simulink model "lqgd_mdl"  (Simulink 5.0)
settings: Solver=ode23s  StartTime=0.0  StopTime=200  RelTol=1e-8  AbsTol=1e-8
values from neighbouring files (symbols this model uses):
  A = [1 -0.9]    [lqg_as1.m]    (also in lqg_ex.m = [1 -0.44]; spec_ex.m = conv([-0.5 1],[-0.9 1]); specfac_ex.m = conv([1 -1],[1 -0.9]))
  B = [0.1 0.08]    [lqg_as1.m]    (also in lqg_ex.m = [0.51 1.21]; lqg_pend.m = num(first_nz:length(num)); spec_ex.m = 0.5*[-0.9 1]; specfac_ex.m)
  C = 1    [lqg_as1.m]    (also in lqg_ex.m = A; lqg_pend.m = A; specfac_ex.m = zeros(1,2))
  Ts = 0.01    [lqg_pend.m]
undefined symbols (not defined in the file or in its folder): R, S, zk
settings Model: Creator=kannanm  LastModifiedBy=kannan  ExtModeAutoUpdateStatusClock=off

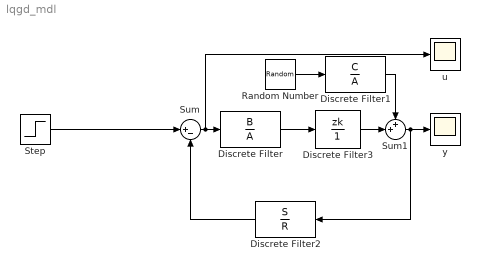
== system lqgd_mdl ==
  Discrete Filter : DiscreteFilter  Numerator=B  Denominator=A  SampleTime=Ts
  Discrete Filter1 : DiscreteFilter  Numerator=C  Denominator=A  SampleTime=Ts
  Discrete Filter2 : DiscreteFilter  Orientation=left  Numerator=S  Denominator=R  SampleTime=Ts
  Discrete Filter3 : DiscreteFilter  Numerator=zk  Denominator=1  SampleTime=Ts
  Random Number : RandomNumber  Variance=0.01  SampleTime=Ts
  Step : Step  After=0  SampleTime=Ts
  Sum : Sum  Inputs=|+-  SaturateOnIntegerOverflow=on
  Sum1 : Sum  Inputs=++|  SaturateOnIntegerOverflow=on
  u : Scope
  y : Scope
  wires:
  Discrete Filter2/1 -> Sum/2
  Discrete Filter/1 -> Discrete Filter3/1
  Sum/1 -> Discrete Filter/1, u/1
  Step/1 -> Sum/1
  Discrete Filter3/1 -> Sum1/2
  Sum1/1 -> y/1, Discrete Filter2/1
  Random Number/1 -> Discrete Filter1/1
  Discrete Filter1/1 -> Sum1/1
